simulink model "third"  (R2023b)
settings: Solver=FixedStepAuto  StartTime=0.0  StopTime=5  FixedStep=0.001  RelTol=1e-3
values from neighbouring files (symbols this model uses):
  A = [-1 0 0 0 ... (first row only)    [untitled.m]    (also in untitled2.m)
  B = [0;1;0;1]    [untitled.m]    (also in untitled2.m)
  K = -Y*pinv(P)    [untitled.m]    (also in untitled2.m)
undefined symbols (not defined in the file or in its folder): C, K1, K2, L, L1, L2, x0, x1
settings Model: Creator=evdokiiagalkina  LastModifiedBy=evdokiiagalkina

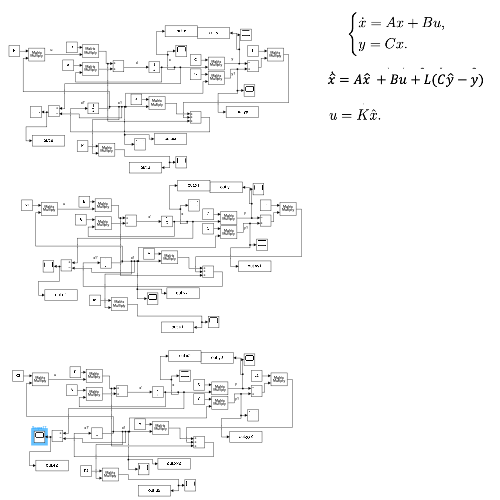
[thumbnail: Simulink's stored preview of the top-level diagram]
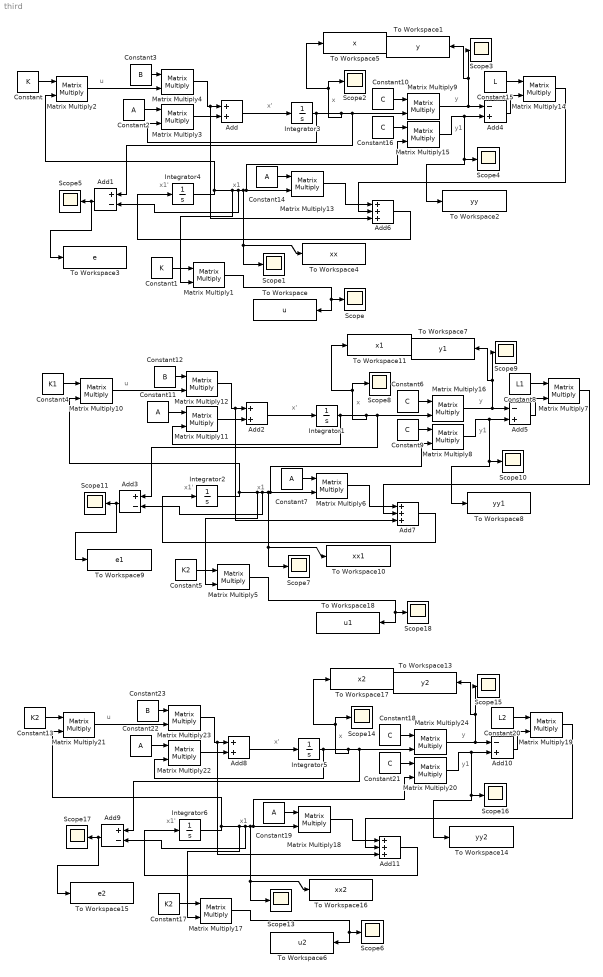
== system third ==
  note: u
  note: y1
  note: y
  note: x'
  note: x
  note: x1
  note: x1'
  note: u
  note: x1
  note: y
  note: x
  note: x1'
  note: y1
  note: x'
  note: u
  note: x1
  note: y
  note: x
  note: x1'
  note: y1
  note: x'
  Add : Sum
  Add1 : Sum  Inputs=+-
  Add10 : Sum  Inputs=-+
  Add11 : Sum  Inputs=+++
  Add2 : Sum
  Add3 : Sum  Inputs=+-
  Add4 : Sum  Inputs=-+
  Add5 : Sum  Inputs=-+
  Add6 : Sum  Inputs=+++
  Add7 : Sum  Inputs=+++
  Add8 : Sum
  Add9 : Sum  Inputs=+-
  Constant : Constant  Value=K  VectorParams1D=off
  Constant1 : Constant  Value=K  VectorParams1D=off
  Constant{6,9..10,16,18,21} (6 alike) : Constant  Value=C  VectorParams1D=off
  Constant{2,7,11,14,19,22} (6 alike) : Constant  Value=A  VectorParams1D=off
  Constant12 : Constant  Value=B  VectorParams1D=off
  Constant13 : Constant  Value=K2  VectorParams1D=off
  Constant15 : Constant  Value=L  VectorParams1D=off
  Constant17 : Constant  Value=K2  VectorParams1D=off
  Constant20 : Constant  Value=L2  VectorParams1D=off
  Constant23 : Constant  Value=B  VectorParams1D=off
  Constant3 : Constant  Value=B  VectorParams1D=off
  Constant4 : Constant  Value=K1  VectorParams1D=off
  Constant5 : Constant  Value=K2  VectorParams1D=off
  Constant8 : Constant  Value=L1  VectorParams1D=off
  Integrator1 : Integrator  InitialCondition=x0
  Integrator2 : Integrator  InitialCondition=x1
  Integrator3 : Integrator  InitialCondition=x0
  Integrator4 : Integrator  InitialCondition=x1
  Integrator5 : Integrator  InitialCondition=x0
  Integrator6 : Integrator  InitialCondition=x1
  Matrix Multiply{1..24} (24 alike) : Product  Multiplication=Matrix(*)
  Scope{,1..11,13..18} (18 alike) : Scope
  To Workspace : ToWorkspace  VariableName=u  SaveFormat=Timeseries  SampleTime=-1
  To Workspace1 : ToWorkspace  VariableName=y  SaveFormat=Timeseries  SampleTime=-1
  To Workspace10 : ToWorkspace  VariableName=xx1  SaveFormat=Timeseries  SampleTime=-1
  To Workspace11 : ToWorkspace  VariableName=x1  SaveFormat=Timeseries  SampleTime=-1
  To Workspace13 : ToWorkspace  VariableName=y2  SaveFormat=Timeseries  SampleTime=-1
  To Workspace14 : ToWorkspace  VariableName=yy2  SaveFormat=Timeseries  SampleTime=-1
  To Workspace15 : ToWorkspace  VariableName=e2  SaveFormat=Timeseries  SampleTime=-1
  To Workspace16 : ToWorkspace  VariableName=xx2  SaveFormat=Timeseries  SampleTime=-1
  To Workspace17 : ToWorkspace  VariableName=x2  SaveFormat=Timeseries  SampleTime=-1
  To Workspace18 : ToWorkspace  VariableName=u1  SaveFormat=Timeseries  SampleTime=-1
  To Workspace2 : ToWorkspace  VariableName=yy  SaveFormat=Timeseries  SampleTime=-1
  To Workspace3 : ToWorkspace  VariableName=e  SaveFormat=Timeseries  SampleTime=-1
  To Workspace4 : ToWorkspace  VariableName=xx  SaveFormat=Timeseries  SampleTime=-1
  To Workspace5 : ToWorkspace  VariableName=x  SaveFormat=Timeseries  SampleTime=-1
  To Workspace6 : ToWorkspace  VariableName=u2  SaveFormat=Timeseries  SampleTime=-1
  To Workspace7 : ToWorkspace  VariableName=y1  SaveFormat=Timeseries  SampleTime=-1
  To Workspace8 : ToWorkspace  VariableName=yy1  SaveFormat=Timeseries  SampleTime=-1
  To Workspace9 : ToWorkspace  VariableName=e1  SaveFormat=Timeseries  SampleTime=-1
  wires:
  Constant10/1 -> Matrix Multiply9/1
  Integrator3/1 -> Matrix Multiply3/2, To Workspace5/1, Scope2/1, Add1/1, Matrix Multiply9/2
  Matrix Multiply9/1 -> Scope3/1, To Workspace1/1, Add4/1
  Add/1 -> Integrator3/1
  Constant14/1 -> Matrix Multiply13/1
  Integrator4/1 -> Matrix Multiply2/2, Add1/2, To Workspace4/1, Scope1/1, Matrix Multiply13/2, Matrix Multiply15/2, Matrix Multiply1/2
  Matrix Multiply13/1 -> Add6/1
  Constant15/1 -> Matrix Multiply14/1
  Add4/1 -> Matrix Multiply14/2
  Matrix Multiply14/1 -> Add6/2
  Add6/1 -> Integrator4/1
  Constant16/1 -> Matrix Multiply15/1
  Matrix Multiply15/1 -> To Workspace2/1, Scope4/1, Add4/2
  Constant1/1 -> Matrix Multiply1/1
  Constant/1 -> Matrix Multiply2/1
  Constant2/1 -> Matrix Multiply3/1
  Matrix Multiply3/1 -> Add/2
  Constant3/1 -> Matrix Multiply4/1
  Matrix Multiply2/1 -> Matrix Multiply4/2
  Matrix Multiply4/1 -> Add6/3, Add/1
  Add1/1 -> To Workspace3/1, Scope5/1
  Add7/1 -> Integrator2/1
  Add3/1 -> To Workspace9/1, Scope11/1
  Matrix Multiply16/1 -> Scope9/1, To Workspace7/1, Add5/1
  Matrix Multiply6/1 -> Add7/1
  Integrator1/1 -> Matrix Multiply11/2, To Workspace11/1, Scope8/1, Add3/1, Matrix Multiply16/2
  Matrix Multiply12/1 -> Add7/3, Add2/1
  Matrix Multiply11/1 -> Add2/2
  Constant4/1 -> Matrix Multiply10/1
  Add5/1 -> Matrix Multiply7/2
  Matrix Multiply7/1 -> Add7/2
  Constant11/1 -> Matrix Multiply11/1
  Integrator2/1 -> Matrix Multiply10/2, Add3/2, To Workspace10/1, Scope7/1, Matrix Multiply6/2, Matrix Multiply8/2, Matrix Multiply5/2
  Constant5/1 -> Matrix Multiply5/1
  Matrix Multiply10/1 -> Matrix Multiply12/2
  Constant12/1 -> Matrix Multiply12/1
  Matrix Multiply8/1 -> To Workspace8/1, Scope10/1, Add5/2
  Constant6/1 -> Matrix Multiply16/1
  Constant7/1 -> Matrix Multiply6/1
  Constant9/1 -> Matrix Multiply8/1
  Add2/1 -> Integrator1/1
  Constant8/1 -> Matrix Multiply7/1
  Add11/1 -> Integrator6/1
  Add9/1 -> To Workspace15/1, Scope17/1
  Matrix Multiply24/1 -> Scope15/1, To Workspace13/1, Add10/1
  Matrix Multiply18/1 -> Add11/1
  Integrator5/1 -> Matrix Multiply22/2, To Workspace17/1, Scope14/1, Add9/1, Matrix Multiply24/2
  Matrix Multiply23/1 -> Add11/3, Add8/1
  Matrix Multiply22/1 -> Add8/2
  Constant13/1 -> Matrix Multiply21/1
  Add10/1 -> Matrix Multiply19/2
  Matrix Multiply19/1 -> Add11/2
  Constant22/1 -> Matrix Multiply22/1
  Integrator6/1 -> Matrix Multiply21/2, Add9/2, To Workspace16/1, Scope13/1, Matrix Multiply18/2, Matrix Multiply20/2, Matrix Multiply17/2
  Constant17/1 -> Matrix Multiply17/1
  Matrix Multiply21/1 -> Matrix Multiply23/2
  Constant23/1 -> Matrix Multiply23/1
  Matrix Multiply20/1 -> To Workspace14/1, Scope16/1, Add10/2
  Constant18/1 -> Matrix Multiply24/1
  Constant19/1 -> Matrix Multiply18/1
  Constant21/1 -> Matrix Multiply20/1
  Add8/1 -> Integrator5/1
  Constant20/1 -> Matrix Multiply19/1
  Matrix Multiply1/1 -> To Workspace/1, Scope/1
  Matrix Multiply5/1 -> To Workspace18/1, Scope18/1
  Matrix Multiply17/1 -> To Workspace6/1, Scope6/1
